simulink model "Loss_3Phase3Level_Inverter"  (Simulink 7.9)
settings: Solver=FixedStepDiscrete  StartTime=0.0  StopTime=12  FixedStep=Ts_Power  RelTol=1e-3
PreLoadFcn:
  | Ts_Power=5e-6
  | Ts_Control=50e-6
undefined symbols (not defined in the file or in its folder): D1, Delta
libraries: powerlib x23, powerlib_extras x21, fl_lib x12, LossModelib x3, nesl_utility x3, simulink x1
settings Model: Creator=Proprietaire  LastModifiedBy=at4494  SimulationMode=accelerator
settings DataIOCC: SaveOutput=off  SaveTime=off
settings OptimizationCC: EfficientMapNaN2IntZero=off
settings HardwareCC: TargetIntDivRoundTo=Zero  TargetEndianess=LittleEndian  TargetHWDeviceType=MATLAB Host  ProdEqTarget=off
settings CodeAppCC: MaxIdLength=128
settings GRTTargetCC: CombineOutputUpdateFcns=off  GRTInterface=on

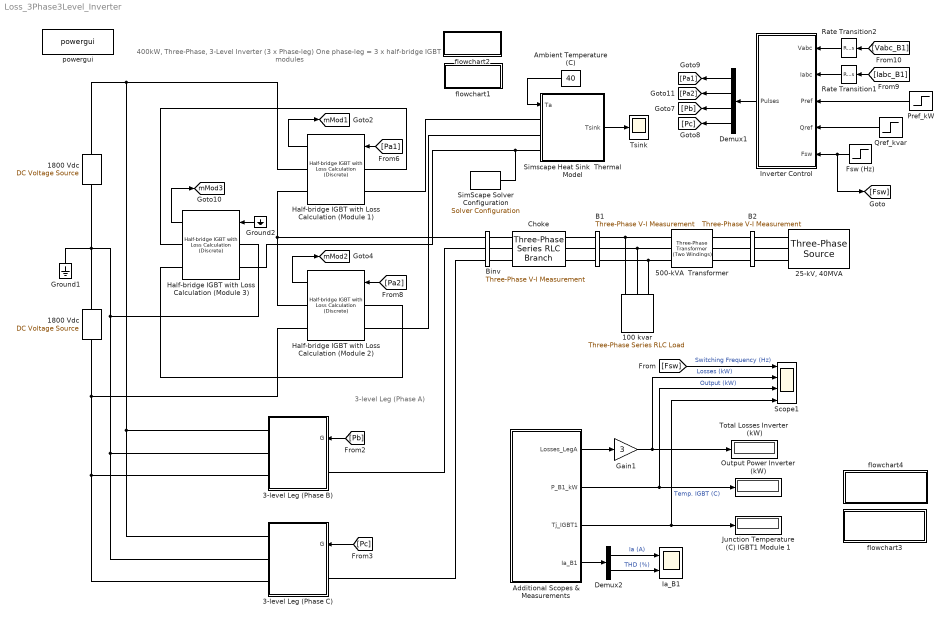
== system Loss_3Phase3Level_Inverter ==
  note: 400kW, Three-Phase, 3-Level Inverter (3 x Phase-leg)
      | One phase-leg = 3 x half-bridge IGBT modules
  note: 3-level Leg
      | (Phase A)
  100 kvar : powerlib/Elements/Three-Phase Series RLC Load  LConnTagsString=A|B|C  Configuration=Y (grounded)  NominalVoltage=2200  NominalFrequency=50  ActivePower=100e3/100  InductivePower=0  CapacitivePower=100e3  Measurements=None  LoadType=constant Z
  1800 Vdc : powerlib/Electrical Sources/DC Voltage Source  Description=source block  Amplitude=1800  Measurements=None
      settings: AttributesFormatString=\n
  "1800 Vdc " : powerlib/Electrical Sources/DC Voltage Source  Description=source block  Amplitude=1800  Measurements=None
      settings: AttributesFormatString=\n
  "25-kV, 40MVA" : powerlib/Electrical Sources/Three-Phase Source  Voltage=25e3*0.99  PhaseAngle=0  Frequency=50  InternalConnection=Yg  SpecifyImpedance=on  Resistance=0.8929  Inductance=16.58e-3  ShortCircuitLevel=40e6  BaseVoltage=25e3  XRratio=7  BusType=swing  Pref=0  Qref=0  Qmin=-inf  Qmax=inf
  3-level Leg (Phase B) : Subsystem
      mask Display:
      | dX=0.02-0.1;
      | dY=0.05-0.34;
      | K=1.4;
      | plot(([0.22 0.292 0.292]+dX)*K,([0.575 0.575 0.685]+dY)*K)
      | %plot([0.19 0.292 0.292]+dX,[0.195 0.195 0.305]+dY)
      | %plot([0.476 0.794]+dX,[0.455 0.455]+dY)
      | plot(([0.476 0.476 0.346 0.346 0.346 0.346 0.476 0.476]+dX)*K,([0.850 0.732 0.680 0.723 0.546 0.622 0.575 0.455 ]+dY)*K)
      | patch(([0.476 0.427 0.415 0.476]+dX)*K,([0.576 0.610 0.576 0.576]+dY)*K)
      | %
      | %plot([0.476 0.476 0.346 0.346 0.346 0.346 0.476 0.476]+dX,[0.850 0.732 0.680 0.723 0.546 0.622 0.575 0.455 ]-0.385+dY)
      | %patch([0.476 0.427 0.415 0.476]+dX,[0.576 0.610 0.576 0.576]-0.385+dY)
      | %
      | plot(([0.614 0.614 0.476]+dX)*K,([0.776 0.507 0.507]+dY)*K)
      | plot(([0.614 0.476]+dX)*K,([0.776 0.776]+dY)*K)
      | plot(([0.577 0.650]+dX)*K,([0.679 0.679]+dY)*K)
      | patch(([0.577 0.650  0.614 0.577]+dX)*K,([0.619 0.619 0.679 0.619]+dY)*K)
      | %
      | %plot([0.614 0.614 0.476]+dX,[0.776 0.507 0.507]-0.385+dY)
      | %plot([0.614 0.476]+dX,[0.776 0.776]-0.385+dY)
      | %plot([0.577 0.650]+dX,[0.679 0.679]-0.385+dY)
      | %patch([0.577 0.650  0.614 0.577]+dX,[0.619 0.619 0.679 0.619]-0.385+dY)
      | %
      | port_label('RConn', 1,'+');
      | port_label('RConn', 2,'N');
      | port_label('RConn', 3,'-');
      | port_label('LConn', 1,'B');
      | color('blue');
      | port_label('input', 1,'G');
  3-level Leg (Phase C) : Subsystem
      mask Display:
      | dX=0.02-0.1;
      | dY=0.05-0.34;
      | K=1.4;
      | plot(([0.22 0.292 0.292]+dX)*K,([0.575 0.575 0.685]+dY)*K)
      | %plot([0.19 0.292 0.292]+dX,[0.195 0.195 0.305]+dY)
      | %plot([0.476 0.794]+dX,[0.455 0.455]+dY)
      | plot(([0.476 0.476 0.346 0.346 0.346 0.346 0.476 0.476]+dX)*K,([0.850 0.732 0.680 0.723 0.546 0.622 0.575 0.455 ]+dY)*K)
      | patch(([0.476 0.427 0.415 0.476]+dX)*K,([0.576 0.610 0.576 0.576]+dY)*K)
      | %
      | %plot([0.476 0.476 0.346 0.346 0.346 0.346 0.476 0.476]+dX,[0.850 0.732 0.680 0.723 0.546 0.622 0.575 0.455 ]-0.385+dY)
      | %patch([0.476 0.427 0.415 0.476]+dX,[0.576 0.610 0.576 0.576]-0.385+dY)
      | %
      | plot(([0.614 0.614 0.476]+dX)*K,([0.776 0.507 0.507]+dY)*K)
      | plot(([0.614 0.476]+dX)*K,([0.776 0.776]+dY)*K)
      | plot(([0.577 0.650]+dX)*K,([0.679 0.679]+dY)*K)
      | patch(([0.577 0.650  0.614 0.577]+dX)*K,([0.619 0.619 0.679 0.619]+dY)*K)
      | %
      | %plot([0.614 0.614 0.476]+dX,[0.776 0.507 0.507]-0.385+dY)
      | %plot([0.614 0.476]+dX,[0.776 0.776]-0.385+dY)
      | %plot([0.577 0.650]+dX,[0.679 0.679]-0.385+dY)
      | %patch([0.577 0.650  0.614 0.577]+dX,[0.619 0.619 0.679 0.619]-0.385+dY)
      | %
      | port_label('RConn', 1,'+');
      | port_label('RConn', 2,'N');
      | port_label('RConn', 3,'-');
      | port_label('LConn', 1,'C');
      | color('blue');
      | port_label('input', 1,'G');
  500-kVA  Transformer : powerlib/Elements/Three-Phase Transformer (Two Windings)  Winding1Connection=Yg  UNITS=pu  NominalPower=[ 500e3 , 50 ]  Winding1=[ 25e3 , 0.001 , 0.025 ]  Winding2Connection=Delta (D1)  Winding2=[ 2200, 0.001 , 0.025 ]  SetSaturation=off  Rm=500  Lm=500  Saturation=[ 0,0 ; 0.0024,1.2 ; 1.0,1.52 ]  Hysteresis=off  DataFile='hysteresis'  SetInitialFlux=off  InitialFluxes=[ 0.8 , -0.8 , 0.7 ]  Measurements=None  MoreParameters=off  BreakLoop=off  DataType=off  TransfoNumber=1
  Additional Scopes & Measurements : Subsystem
  Ambient Temperature (C) : Constant  Value=40
  B1 : powerlib/Measurements/Three-Phase V-I Measurement  VoltageMeasurement=phase-to-ground  SetLabelV=on  LabelV=Vabc_B1  Vpu=off  VpuLL=off  CurrentMeasurement=yes  SetLabelI=on  LabelI=Iabc_B1  Ipu=off  Pbase=100e6  Vbase=500e3  OutputType=Complex  PhasorSimulation=off  PSBequivalent=0
  B2 : powerlib/Measurements/Three-Phase V-I Measurement  VoltageMeasurement=phase-to-ground  SetLabelV=on  LabelV=Vabc_B2  Vpu=off  VpuLL=off  CurrentMeasurement=yes  SetLabelI=on  LabelI=Iabc_B2  Ipu=off  Pbase=100e6  Vbase=500e3  OutputType=Complex  PhasorSimulation=off  PSBequivalent=0
  Binv : powerlib/Measurements/Three-Phase V-I Measurement  VoltageMeasurement=phase-to-ground  SetLabelV=on  LabelV=Vabc_Binv  Vpu=off  VpuLL=off  CurrentMeasurement=yes  SetLabelI=on  LabelI=Iabc_Binv  Ipu=off  Pbase=100e6  Vbase=500e3  OutputType=Complex  PhasorSimulation=off  PSBequivalent=0
  Choke : powerlib/Elements/Three-Phase Series RLC Branch  LConnTagsString=A|B|C  RConnTagsString=A|B|C  BranchType=RL  Resistance=15e-3  Inductance=5e-3  Capacitance=1e-6  Measurements=None
  Demux1 : Demux  Outputs=[ 2 2 4 4 ]
  Demux2 : Demux  Outputs=2
  Fsw (Hz) : Step  Time=5  Before=17*50  After=37*50  SampleTime=Ts_Control
  Gain1 : Gain  Gain=3
  Ground1 : powerlib/Elements/Ground  LConnTagsString=a
  Ground2 : Ground
  Half-bridge IGBT with Loss Calculation (Module 1) : LossModelib/Half-bridge IGBT with Loss Calculation (Discrete)  Ron=1e-3  IGBT_Type=ABB: Half-Bridge IGBT 3300V/250A  PlotSpec_IGBT_On=off  ShowDataSheet_IGBT_On=off  Diode_Type=ABB: Half-Bridge IGBT 3300V/250A  PlotSpec_Diode_On=off  ShowDataSheet_Diode_On=off  Tj_Init=123  PulseDuration=5e-6  Ts_Simscape=Ts_Control  Ts=Ts_Power
  Half-bridge IGBT with Loss Calculation (Module 2) : LossModelib/Half-bridge IGBT with Loss Calculation (Discrete)  Ron=1e-3  IGBT_Type=ABB: Half-Bridge IGBT 3300V/250A  PlotSpec_IGBT_On=off  ShowDataSheet_IGBT_On=off  Diode_Type=ABB: Half-Bridge IGBT 3300V/250A  PlotSpec_Diode_On=off  ShowDataSheet_Diode_On=off  Tj_Init=123  PulseDuration=5e-6  Ts_Simscape=Ts_Control  Ts=Ts_Power
  Half-bridge IGBT with Loss Calculation (Module 3) : LossModelib/Half-bridge IGBT with Loss Calculation (Discrete)  Ron=1e-3  IGBT_Type=ABB: Half-Bridge IGBT 3300V/250A  PlotSpec_IGBT_On=off  ShowDataSheet_IGBT_On=off  Diode_Type=ABB: Half-Bridge IGBT 3300V/250A  PlotSpec_Diode_On=off  ShowDataSheet_Diode_On=off  Tj_Init=123  PulseDuration=5e-6  Ts_Simscape=Ts_Control  Ts=Ts_Power
  Ia_B1 : Scope  NumInputPorts=2
      settings: TimeRange=12  YMin=-300~10  YMax=300~30  SaveName=psb1phPWM2_str3  MaxDataPoints=500000
  Inverter Control : Subsystem  mask(Inverter Control         ){nom=[ 500e3  50 ], Vnom=2200, Vnom_dc=2*1800, RLchoke=[15e-3  5e-3  ], K_PQreg=[ 0.2  60 ], K_Ireg=[0.3 20], Ts=Ts_Control}
      mask prompts: nom "Nominal power and frequency [ Pnom(VA)  Fnom(Hz) ]:"; Vnom "Nominal voltage (Vrms LL):"; Vnom_dc "Nominal DC bus voltage (V):"; RLchoke "Choke impedance [ R(ohm) L(H) ]"; K_PQreg "PQ regulator gains [ Kp  Ki ]:"; K_Ireg "Current regulator gains [ Kp  Ki ]:"; Ts "Sample time"
      mask init:
      | Pnom=nom(1);
      | Fnom=nom(2);
      | Zbase=Vnom^2/Pnom;
      | Rtot_pu= RLchoke(1)/Zbase;
      | Ltot_pu= RLchoke(2)/(Zbase/(2*pi*Fnom));
      | Kp_PQreg=K_PQreg(1);
      | Ki_PQreg=K_PQreg(2);
      | Kp_Ireg=K_Ireg(1);
      | Ki_Ireg=K_Ireg(2);
      | Vdc_ref=Vnom_dc;
  Junction Temperature (C) IGBT1 Module 1 : Display
      settings: Format=bank  Decimation=1000
  Output Power Inverter (kW) : Display
      settings: Format=bank  Decimation=1000
  Pref_kW : Step  Time=5.1  Before=372  After=211  SampleTime=Ts_Control
  Qref_kvar : Step  Time=5.1  Before=-sqrt(372^2*(1/(0.85)^2 - 1))  After=-sqrt(211^2*(1/(0.85)^2 - 1))  SampleTime=Ts_Control
  Rate Transition1 : RateTransition  OutPortSampleTime=Ts_Control
  Rate Transition2 : RateTransition  OutPortSampleTime=Ts_Control
  Scope1 : Scope  NumInputPorts=4
      settings: TimeRange=12  YMin=600~2~100~115  YMax=2000~4~500~135  SaveName=psb1phPWM2_str1  MaxDataPoints=500000  Decimation=10
  SimScape Solver Configuration : nesl_utility/Solver Configuration  PhysicalDomain=network_engine_domain  LeftPortType=input  RightPortType=generic  SubClassName=solver  UseCustomDae=off  DoDC=off  ResidualTolerance=1e-9  UseLocalSolver=on  LocalSolverChoice=NE_TRAPEZOIDAL_ADVANCER  LocalSolverSampleTime=Ts_Control  DoFixedCost=off  MaxNonlinIter=2  MaxModeIter=1  LinearAlgebra=Sparse  Accelerate=off  Profile=off  UseLocalSampling=off  DelaysMemoryBudget=1024
  Simscape Heat Sink  Thermal Model : Subsystem  mask(Simscape Thermal model (2-cell Cauer network)){Rth=[ 0.02  0.072 ], Cth=[ 1  5 ]/10, Tinit=123}
      mask prompts: Rth "Thermal resistances  [case-to-sink  sink-to-ambient ] (K/W):"; Cth "Thermal capacitances  [case  sink ] (J/K):"; Tinit "Initial temperature (degrees Celsisus)"
  Total Losses Inverter (kW) : Display
      settings: Format=bank  Decimation=1000
  Tsink : Scope
      settings: TimeRange=12  YMin=101.4492375546095  YMax=109.4893107691547  SaveName=psb1phPWM2_str6  MaxDataPoints=500000  Decimation=100
  flowchart1 : Subsystem
      settings: OpenFcn=winopen('ABB_PhaseLegModule_PCIM_12_408.pdf');
      mask Display: disp('Reference\nDocument')
  flowchart2 : Subsystem
      settings: OpenFcn=winopen('Loss_3Phase3Level_Inverter_Help.pdf');
      mask Display: disp('Help')
  flowchart3 : Subsystem
      settings: OpenFcn=plot_FFTresults
      mask Display: disp('Plot\nFFT Comparison')
  flowchart4 : Subsystem
      settings: OpenFcn=plot_OutputPower_vs_SwitchingFrequency
      mask Display: disp('Plot\n OutputPower vs.\nSwitching Frequency')
  powergui : powerlib/powergui  Priority=1  SimulationMode=Discrete  SolverType=Tustin  SampleTime=Ts_Power  frequency=60  SPID=off  DisableSnubberDevices=off  DisableRonSwitches=off  DisableVfSwitches=off  SwTol=0  Interpol=off  DisplayEquations=off  FunctionMessages=off  frequencyindice=0  Pbase=100e6  ErrMax=1e-4  Iterations=50  UnitsV=kV  UnitsW=MW  echomessages=off  HookPort=off  EnableUseOfTLC=off  x0status=blocks  RestoreLinks=warning  ResistiveCurrentMeasurement=off  Ylog=off  Xlog=on  ShowGrid=off  save=off  variable=ZData  structure=VIabc_B1  ZoomFFT=off  StartTime=4  cycles=3  DisplayStyle=1  fundamental=50  FreqAxis=on  MaxFrequency=2500  frequencyindicesteady=1  display=off  methode=off
  tag scope: mMod1=global, mMod2=global, mMod3=global
  wires:
  [Pb] -> 3-level Leg (Phase B)/1(G)
  Ambient Temperature (C)/1 -> Simscape Heat Sink  Thermal Model/1(Ta)
  [Pc] -> 3-level Leg (Phase C)/1(G)
  Additional Scopes & Measurements/1(Losses_LegA) -> Gain1/1
  [Vabc_B1] -> Rate Transition2/1
  [Iabc_B1] -> Rate Transition1/1
  Demux1/1 -> [Pa1]
  Demux1/2 -> [Pa2]
  Demux1/4 -> [Pc]
  Demux1/3 -> [Pb]
  Inverter Control/1(Pulses) -> Demux1/1
  Pref_kW/1 -> Inverter Control/3(Pref)
  Qref_kvar/1 -> Inverter Control/4(Qref)
  Additional Scopes & Measurements/2(P_B1_kW) -> Output Power Inverter (kW)/1, Scope1/3  "Output (kW)"
  Fsw (Hz)/1 -> Inverter Control/5(Fsw), [Fsw]
  Rate Transition1/1 -> Inverter Control/2(Iabc)
  Rate Transition2/1 -> Inverter Control/1(Vabc)
  Simscape Heat Sink  Thermal Model/1(Tsink) -> Tsink/1
  Half-bridge IGBT with Loss Calculation (Module 3)/1 -> [mMod3]
  Half-bridge IGBT with Loss Calculation (Module 2)/1 -> [mMod2]
  Ground2/1 -> Half-bridge IGBT with Loss Calculation (Module 3)/1
  [Pa1] -> Half-bridge IGBT with Loss Calculation (Module 1)/1
  [Pa2] -> Half-bridge IGBT with Loss Calculation (Module 2)/1
  Half-bridge IGBT with Loss Calculation (Module 1)/1 -> [mMod1]
  Additional Scopes & Measurements/3(Tj_IGBT1) -> Junction Temperature (C) IGBT1 Module 1/1, Scope1/4  "Temp. IGBT (C)"
  Gain1/1 -> Total Losses Inverter (kW)/1, Scope1/2  "Losses (kW)"
  [Fsw] -> Scope1/1  "Switching Frequency (Hz)"
  Demux2/1 -> Ia_B1/1  "Ia (A)"
  Demux2/2 -> Ia_B1/2  "THD (%)"
  Additional Scopes & Measurements/4(Ia_B1) -> Demux2/1
  connections:
  Half-bridge IGBT with Loss Calculation (Module 3)/LConn2 -- SimScape Solver Configuration/RConn1 -- Simscape Heat Sink  Thermal Model/LConn3
  Choke/RConn1 -- B1/LConn1
  Choke/RConn2 -- B1/LConn2
  Choke/RConn3 -- B1/LConn3
  "25-kV, 40MVA"/RConn1 -- B2/RConn1
  "25-kV, 40MVA"/RConn2 -- B2/RConn2
  "25-kV, 40MVA"/RConn3 -- B2/RConn3
  Choke/LConn1 -- Binv/RConn1
  Choke/LConn2 -- Binv/RConn2
  Choke/LConn3 -- Binv/RConn3
  Binv/LConn2 -- 3-level Leg (Phase B)/LConn1
  Binv/LConn3 -- 3-level Leg (Phase C)/LConn1
  500-kVA  Transformer/RConn1 -- B1/RConn1 -- 100 kvar/LConn1
  500-kVA  Transformer/RConn2 -- B1/RConn2 -- 100 kvar/LConn2
  B1/RConn3 -- 500-kVA  Transformer/RConn3 -- 100 kvar/LConn3
  500-kVA  Transformer/LConn1 -- B2/LConn1
  500-kVA  Transformer/LConn2 -- B2/LConn2
  500-kVA  Transformer/LConn3 -- B2/LConn3
  Half-bridge IGBT with Loss Calculation (Module 1)/RConn2 -- Binv/LConn1 -- Half-bridge IGBT with Loss Calculation (Module 2)/RConn1
  Half-bridge IGBT with Loss Calculation (Module 3)/LConn1 -- 3-level Leg (Phase B)/RConn2 -- 3-level Leg (Phase C)/RConn2 -- 1800 Vdc/RConn1 -- Ground1/LConn1 -- "1800 Vdc "/LConn1
  Simscape Heat Sink  Thermal Model/LConn1 -- Half-bridge IGBT with Loss Calculation (Module 1)/LConn2
  Half-bridge IGBT with Loss Calculation (Module 1)/RConn1 -- 3-level Leg (Phase B)/RConn1 -- 3-level Leg (Phase C)/RConn1 -- "1800 Vdc "/RConn1
  Half-bridge IGBT with Loss Calculation (Module 2)/RConn2 -- 3-level Leg (Phase B)/RConn3 -- 3-level Leg (Phase C)/RConn3 -- 1800 Vdc/LConn1
  Half-bridge IGBT with Loss Calculation (Module 3)/RConn1 -- Half-bridge IGBT with Loss Calculation (Module 1)/LConn1
  Half-bridge IGBT with Loss Calculation (Module 2)/LConn1 -- Half-bridge IGBT with Loss Calculation (Module 3)/RConn2
  Half-bridge IGBT with Loss Calculation (Module 2)/LConn2 -- Simscape Heat Sink  Thermal Model/LConn2

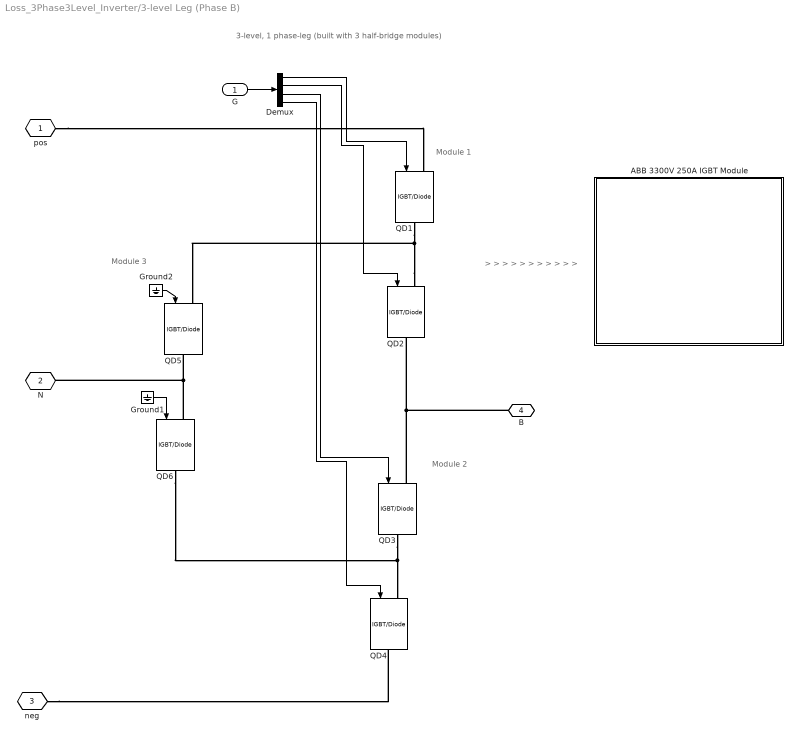
== system Loss_3Phase3Level_Inverter/3-level Leg (Phase B) ==
  note: Module 3
  note: Module 2
  note: 3-level, 1 phase-leg
      |  (built with 3 half-bridge modules)
  note: Module 1
  note: > > > > > > > > > > >
  G : Inport  PortDimensions=4
  ABB 3300V 250A IGBT Module : Subsystem
      mask Display: image(imread('Picture_IGBT_Module.jpg'))
  Demux : Demux
  Ground1 : Ground
  Ground2 : Ground
  QD{1..6} (6 alike) : powerlib/Power Electronics/IGBT//Diode  Ron=1e-3  Rs=1e5  Cs=inf  Measurements=off
  pos : PMIOPort  Port=1  Side=Right
  N : PMIOPort  Port=2  Side=Right
  neg : PMIOPort  Port=3  Side=Right
  B : PMIOPort  Port=4  Side=Left
  wires:
  Demux/4 -> QD4/1
  Demux/3 -> QD3/1
  Ground1/1 -> QD6/1
  Ground2/1 -> QD5/1
  G/1 -> Demux/1
  Demux/1 -> QD1/1
  Demux/2 -> QD2/1
  connections:
  N/RConn1 -- QD6/LConn1 -- QD5/RConn1
  QD3/RConn1 -- QD4/LConn1 -- QD6/RConn1
  QD2/LConn1 -- QD1/RConn1 -- QD5/LConn1
  pos/RConn1 -- QD1/LConn1
  QD3/LConn1 -- QD2/RConn1 -- B/RConn1
  neg/RConn1 -- QD4/RConn1

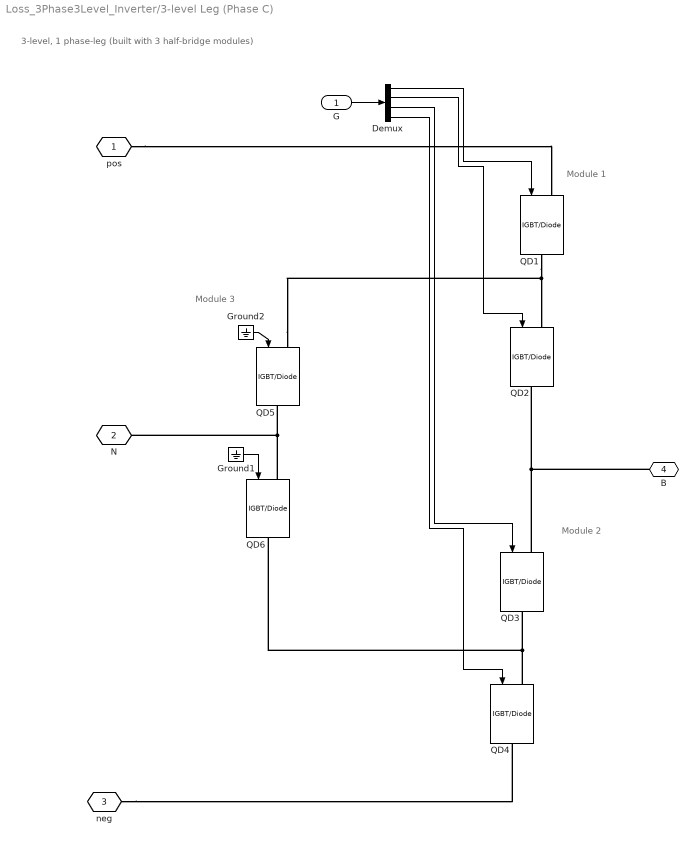
== system Loss_3Phase3Level_Inverter/3-level Leg (Phase C) ==
  note: Module 1
  note: 3-level, 1 phase-leg
      |  (built with 3 half-bridge modules)
  note: Module 2
  note: Module 3
  G : Inport  PortDimensions=4
  Demux : Demux
  Ground1 : Ground
  Ground2 : Ground
  QD{1..6} (6 alike) : powerlib/Power Electronics/IGBT//Diode  Ron=1e-3  Rs=1e5  Cs=inf  Measurements=off
  pos : PMIOPort  Port=1  Side=Right
  N : PMIOPort  Port=2  Side=Right
  neg : PMIOPort  Port=3  Side=Right
  B : PMIOPort  Port=4  Side=Left
  wires:
  Demux/2 -> QD2/1
  Demux/1 -> QD1/1
  G/1 -> Demux/1
  Ground2/1 -> QD5/1
  Ground1/1 -> QD6/1
  Demux/3 -> QD3/1
  Demux/4 -> QD4/1
  connections:
  neg/RConn1 -- QD4/RConn1
  B/RConn1 -- QD2/RConn1 -- QD3/LConn1
  pos/RConn1 -- QD1/LConn1
  QD5/LConn1 -- QD2/LConn1 -- QD1/RConn1
  QD4/LConn1 -- QD3/RConn1 -- QD6/RConn1
  QD6/LConn1 -- N/RConn1 -- QD5/RConn1

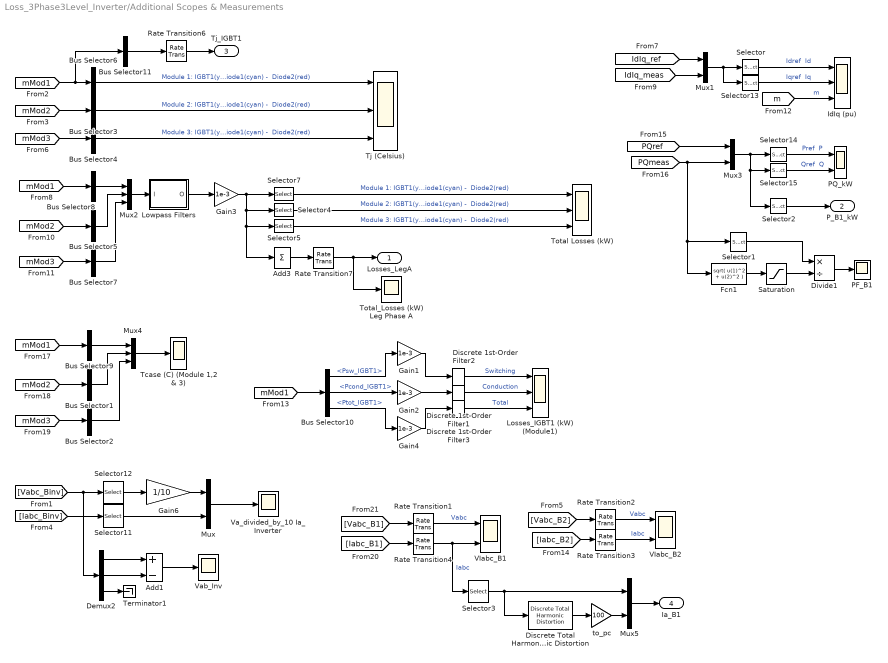
== system Loss_3Phase3Level_Inverter/Additional Scopes & Measurements ==
  Add1 : Sum  Inputs=+-
  Add3 : Sum  Inputs=+
  Bus Selector1 : BusSelector  OutputSignals=Tcase  OutputAsBus=on
  Bus Selector10 : BusSelector  OutputSignals=Psw_IGBT1,Pcond_IGBT1,Ptot_IGBT1
  Bus Selector11 : BusSelector  OutputSignals=Tj_IGBT1  OutputAsBus=on
  Bus Selector2 : BusSelector  OutputSignals=Tcase  OutputAsBus=on
  Bus Selector3 : BusSelector  OutputSignals=Tj_IGBT1,Tj_IGBT2,Tj_Diode1,Tj_Diode2  OutputAsBus=on
  Bus Selector4 : BusSelector  OutputSignals=Tj_IGBT1,Tj_IGBT2,Tj_Diode1,Tj_Diode2  OutputAsBus=on
  Bus Selector5 : BusSelector  OutputSignals=Ptot_IGBT1,Ptot_IGBT2,Ptot_Diode1,Ptot_Diode2  OutputAsBus=on
  Bus Selector6 : BusSelector  OutputSignals=Tj_IGBT1,Tj_IGBT2,Tj_Diode1,Tj_Diode2  OutputAsBus=on
  Bus Selector7 : BusSelector  OutputSignals=Ptot_IGBT1,Ptot_IGBT2,Ptot_Diode1,Ptot_Diode2  OutputAsBus=on
  Bus Selector8 : BusSelector  OutputSignals=Ptot_IGBT1,Ptot_IGBT2,Ptot_Diode1,Ptot_Diode2  OutputAsBus=on
  Bus Selector9 : BusSelector  OutputSignals=Tcase  OutputAsBus=on
  Demux2 : Demux  Outputs=3
  Discrete 1st-Order Filter1 : powerlib_extras/Discrete  Control Blocks/Discrete 1st-Order Filter  FilterType=Lowpass  Tc=100e-3  Ts=Ts_Power  Initialize=off  Vac_Init=[0.8 -25 60]  Vdc_Init=-0.4  PlotResponse=off  param1=[1 500 0.1]
  Discrete 1st-Order Filter2 : powerlib_extras/Discrete  Control Blocks/Discrete 1st-Order Filter  FilterType=Lowpass  Tc=100e-3  Ts=Ts_Power  Initialize=off  Vac_Init=[0.8 -25 60]  Vdc_Init=-0.4  PlotResponse=off  param1=[1 500 0.1]
  Discrete 1st-Order Filter3 : powerlib_extras/Discrete  Control Blocks/Discrete 1st-Order Filter  FilterType=Lowpass  Tc=100e-3  Ts=Ts_Power  Initialize=off  Vac_Init=[0.8 -25 60]  Vdc_Init=-0.4  PlotResponse=off  param1=[1 500 0.1]
  Discrete Total Harmonic Distortion : powerlib_extras/Discrete Measurements/Discrete Total Harmonic Distortion  Freq=50  Ts=Ts_Control
  Divide1 : Product  Inputs=*/
  Fcn1 : Fcn  Expr=sqrt( u(1)^2 + u(2)^2 )
  Gain{1..4} (4 alike) : Gain  Gain=1e-3
  Gain6 : Gain  Gain=1/10
  IdIq (pu) : Scope  NumInputPorts=3
      settings: TimeRange=12  YMin=0~0~0.7000000000000001  YMax=1.4~1.4~1.2  SaveName=Vab_Load  MaxDataPoints=500000
  Losses_IGBT1 (kW) (Module1) : Scope  NumInputPorts=3
      settings: TimeRange=12  YMin=0~0~0  YMax=0.4~0.1~0.4  SaveName=Va_Load  MaxDataPoints=500000  Decimation=100
  Lowpass Filters : Subsystem  mask(12 x First-Order Lowpass Filters){Tc=100e-3, Ts=Ts_Power}
      mask prompts: Tc "Time constant (s):"; Ts "Sample time (s):"
  Mux : Mux  Inputs=2
  Mux1 : Mux  Inputs="[ 2  2 ]"
  Mux2 : Mux  Inputs=3
  Mux3 : Mux  Inputs="[ 2  2 ]"
  Mux4 : Mux  Inputs=3
  Mux5 : Mux  Inputs=2
  PF_B1 : Scope
      settings: TimeRange=12  YMin=0.8180348878604487  YMax=0.8857030971876113  SaveName=Va_Load5  MaxDataPoints=500000
  PQ_kW : Scope  NumInputPorts=2
      settings: TimeRange=12  YMin=0~-400  YMax=500~100  SaveName=Vab_Load2  MaxDataPoints=500000
  Rate Transition{1..4,6..7} (6 alike) : RateTransition  OutPortSampleTime=Ts_Control
  Saturation : Saturate  UpperLimit=inf  LowerLimit=eps
  Selector : Selector  InputPortWidth=4  IndexOptions=Index vector (dialog)  Indices=[1 3]  OutputSizes=1
  Selector1 : Selector  InputPortWidth=2  IndexOptions=Index vector (dialog)  Indices=[1]  OutputSizes=1
  Selector11 : Selector  InputPortWidth=3  IndexOptions=Index vector (dialog)  Indices=[1]  OutputSizes=1
  Selector12 : Selector  InputPortWidth=3  IndexOptions=Index vector (dialog)  Indices=[1]  OutputSizes=1
  Selector13 : Selector  InputPortWidth=4  IndexOptions=Index vector (dialog)  Indices=[1 3]  OutputSizes=1
  Selector14 : Selector  InputPortWidth=4  IndexOptions=Index vector (dialog)  Indices=[1 3]  OutputSizes=1
  Selector15 : Selector  InputPortWidth=4  IndexOptions=Index vector (dialog)  Indices=[2 4]  OutputSizes=1
  Selector2 : Selector  InputPortWidth=4  IndexOptions=Index vector (dialog)  Indices=[3]  OutputSizes=1
  Selector3 : Selector  InputPortWidth=3  IndexOptions=Index vector (dialog)  Indices=[1]  OutputSizes=1
  Selector4 : Selector  InputPortWidth=12  IndexOptions=Index vector (dialog)  Indices=[1 2 3 4]+4  OutputSizes=1
  Selector5 : Selector  InputPortWidth=12  IndexOptions=Index vector (dialog)  Indices=[1 2 3 4]+8  OutputSizes=1
  Selector7 : Selector  InputPortWidth=12  IndexOptions=Index vector (dialog)  Indices=[1 2 3 4]  OutputSizes=1
  Tcase (C) (Module 1,2 & 3) : Scope
      settings: TimeRange=12  YMin=100  YMax=120  SaveName=psb1phPWM2_str2  MaxDataPoints=500000  Decimation=100
  Terminator1 : Terminator
  Tj (Celsius) : Scope  NumInputPorts=3
      settings: TimeRange=12  YMin=105~105~105  YMax=135~135~135  SaveName=psb1phPWM2_str  MaxDataPoints=500000  Decimation=100
  "Total Losses (kW) " : Scope  NumInputPorts=3
      settings: TimeRange=12  YMin=0~0~0  YMax=0.4~0.4~0.14  SaveName=Losses_Scope  MaxDataPoints=500000  Decimation=100
  Total_Losses (kW) Leg Phase A : Scope
      settings: TimeRange=12  YMin=0  YMax=1.4  SaveName=Va_Load6  MaxDataPoints=500000  Decimation=10
  VIabc_B1 : Scope  NumInputPorts=2
      settings: TimeRange=12  YMin=-2500~-504.4510385756676  YMax=2500~459.9406528189911  SaveName=VIabc_B1  MaxDataPoints=500000
  VIabc_B2 : Scope  NumInputPorts=2
      settings: YMin=-25000~-20  YMax=25000~25  SaveName=VIabc_B2  MaxDataPoints=500000
  Va_divided_by_10 Ia_Inverter : Scope
      settings: YMin=-500  YMax=500  SaveName=psb1phPWM2_str5  MaxDataPoints=500000  Decimation=2
  Vab_Inv : Scope
      settings: TimeRange=0.08  YMin=-4000  YMax=4000  SaveName=Vab_Inv  MaxDataPoints=500000  Decimation=2
  to_pc : Gain  Gain=100
  Losses_LegA : Outport
  P_B1_kW : Outport  Port=2
  Tj_IGBT1 : Outport  Port=3
  Ia_B1 : Outport  Port=4
  wires:
  Mux/1 -> Va_divided_by_10 Ia_Inverter/1
  [mMod1] -> Bus Selector6/1, Bus Selector11/1
  [mMod2] -> Bus Selector3/1
  [mMod3] -> Bus Selector4/1
  [mMod1] -> Bus Selector8/1
  [mMod2] -> Bus Selector5/1
  [mMod3] -> Bus Selector7/1
  Mux2/1 -> Lowpass Filters/1(I)
  Selector7/1 -> "Total Losses (kW) "/1  "Module 1: IGBT1(yellow) -  IGBT2(magenta)  -  Diode1(cyan) -  Diode2(red)"
  Selector4/1 -> "Total Losses (kW) "/2  "Module 2: IGBT1(yellow) -  IGBT2(magenta)  -  Diode1(cyan) -  Diode2(red)"
  Selector5/1 -> "Total Losses (kW) "/3  "Module 3: IGBT1(yellow) -  IGBT2(magenta)  -  Diode1(cyan) -  Diode2(red)"
  Bus Selector8/1 -> Mux2/1
  Bus Selector5/1 -> Mux2/2
  Bus Selector7/1 -> Mux2/3
  Lowpass Filters/1(O) -> Gain3/1
  Gain3/1 -> Selector7/1, Add3/1, Selector5/1, Selector4/1
  Add3/1 -> Rate Transition7/1
  [Vabc_Binv] -> Selector12/1, Demux2/1
  [Iabc_Binv] -> Selector11/1
  Selector12/1 -> Gain6/1
  Selector11/1 -> Mux/2
  Gain6/1 -> Mux/1
  Fcn1/1 -> Saturation/1
  Selector1/1 -> Divide1/1
  Divide1/1 -> PF_B1/1
  [IdIq_ref] -> Mux1/1
  Saturation/1 -> Divide1/2
  Demux2/1 -> Add1/1
  Demux2/2 -> Add1/2
  Demux2/3 -> Terminator1/1
  Add1/1 -> Vab_Inv/1
  [mMod1] -> Bus Selector9/1
  [mMod2] -> Bus Selector1/1
  [mMod3] -> Bus Selector2/1
  Bus Selector9/1 -> Mux4/1
  Bus Selector1/1 -> Mux4/2
  Bus Selector2/1 -> Mux4/3
  Mux4/1 -> Tcase (C) (Module 1,2 & 3)/1
  [m] -> IdIq (pu)/3  "m"
  [IdIq_meas] -> Mux1/2
  Mux1/1 -> Selector/1, Selector13/1
  Selector/1 -> IdIq (pu)/1  "Idref  Id"
  Selector13/1 -> IdIq (pu)/2  "Iqref  Iq"
  [PQref] -> Mux3/1
  [PQmeas] -> Mux3/2, Selector1/1, Fcn1/1
  Mux3/1 -> Selector14/1, Selector15/1, Selector2/1
  Selector14/1 -> PQ_kW/1  "Pref  P"
  Selector15/1 -> PQ_kW/2  "Qref  Q"
  Selector2/1 -> P_B1_kW/1
  [Vabc_B1] -> Rate Transition1/1
  [Iabc_B1] -> Rate Transition4/1
  Rate Transition1/1 -> VIabc_B1/1  "Vabc"
  Rate Transition4/1 -> VIabc_B1/2, Selector3/1  "Iabc"
  [mMod1] -> Bus Selector10/1
  Bus Selector10/1 -> Gain1/1  "<Psw_IGBT1>"
  Bus Selector10/2 -> Gain2/1  "<Pcond_IGBT1>"
  Bus Selector10/3 -> Gain4/1  "<Ptot_IGBT1>"
  Discrete 1st-Order Filter2/1 -> Losses_IGBT1 (kW) (Module1)/1  "Switching"
  Rate Transition2/1 -> VIabc_B2/1  "Vabc"
  Rate Transition3/1 -> VIabc_B2/2  "Iabc"
  [Vabc_B2] -> Rate Transition2/1
  [Iabc_B2] -> Rate Transition3/1
  Bus Selector6/1 -> Tj (Celsius)/1  "Module 1: IGBT1(yellow) -  IGBT2(magenta)  -  Diode1(cyan) -  Diode2(red)"
  Bus Selector3/1 -> Tj (Celsius)/2  "Module 2: IGBT1(yellow) -  IGBT2(magenta)  -  Diode1(cyan) -  Diode2(red)"
  Bus Selector4/1 -> Tj (Celsius)/3  "Module 3: IGBT1(yellow) -  IGBT2(magenta)  -  Diode1(cyan) -  Diode2(red)"
  Discrete 1st-Order Filter1/1 -> Losses_IGBT1 (kW) (Module1)/2  "Conduction"
  Discrete 1st-Order Filter3/1 -> Losses_IGBT1 (kW) (Module1)/3  "Total"
  Gain1/1 -> Discrete 1st-Order Filter2/1
  Gain2/1 -> Discrete 1st-Order Filter1/1
  Gain4/1 -> Discrete 1st-Order Filter3/1
  Rate Transition6/1 -> Tj_IGBT1/1
  Bus Selector11/1 -> Rate Transition6/1
  Rate Transition7/1 -> Losses_LegA/1, Total_Losses (kW) Leg Phase A/1
  Discrete Total Harmonic Distortion/1 -> to_pc/1
  Selector3/1 -> Mux5/1, Discrete Total Harmonic Distortion/1
  Mux5/1 -> Ia_B1/1
  to_pc/1 -> Mux5/2

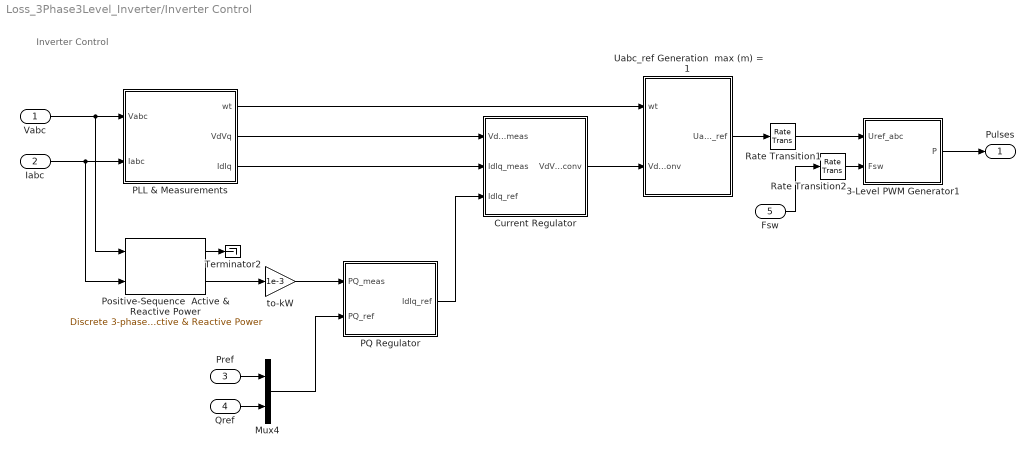
== system Loss_3Phase3Level_Inverter/Inverter Control ==
  note: Inverter Control
  Vabc : Inport  PortDimensions=3  SampleTime=Ts
  Iabc : Inport  Port=2  PortDimensions=3  SampleTime=Ts
  Pref : Inport  Port=3  PortDimensions=1  SampleTime=Ts
  Qref : Inport  Port=4  PortDimensions=1  SampleTime=Ts
  Fsw : Inport  Port=5  PortDimensions=1
  " Positive-Sequence  Active & Reactive Power" : powerlib_extras/Discrete Measurements/Discrete 3-phase  Positive-Sequence  Active & Reactive Power  Freq=Fnom  Par_Vinit=[100 10]  Par_Iinit=[1 1]  Ts=Ts
  3-Level PWM Generator1 : Subsystem  mask(Discrete 3-Phase, 3-Level, PWM Generator){Ts=Ts_Power}
      mask prompts: Ts "Sample time (s):"
      mask help:
      | Generate pulses for carrier-based Pulse Width Modulation (PWM) 3-Level, 3-Phase converters.
      | Input 1: Three-phase reference signals (Uref_abc)
      | Input 2: Switching frequency (Fsw)
      | Output: Vectorized output P contains the 12 pulses.  Look Under Mask to get a description of the pulse pattern.
  Current Regulator : Subsystem
  Mux4 : Mux  Inputs=2
  PLL & Measurements : Subsystem
  PQ Regulator : Subsystem
  Rate Transition1 : RateTransition  OutPortSampleTime=Ts_Power
  Rate Transition2 : RateTransition  OutPortSampleTime=Ts_Power
  Terminator2 : Terminator
  Uabc_ref Generation  max (m) = 1 : Subsystem
  to-kW : Gain  Gain=1e-3  SaturateOnIntegerOverflow=on  OutDataTypeStr=Inherit: Same as input  ParamDataTypeStr=Inherit: Same as input
  Pulses : Outport
  wires:
  Uabc_ref Generation  max (m) = 1/1(Uabc_ref) -> Rate Transition1/1
  Iabc/1 -> PLL & Measurements/2(Iabc), " Positive-Sequence  Active & Reactive Power"/2
  Vabc/1 -> PLL & Measurements/1(Vabc), " Positive-Sequence  Active & Reactive Power"/1
  PLL & Measurements/2(VdVq) -> Current Regulator/1(VdVq_meas)
  PLL & Measurements/3(IdIq) -> Current Regulator/2(IdIq_meas)
  Current Regulator/1(VdVq_conv) -> Uabc_ref Generation  max (m) = 1/2(VdVq_conv)
  PLL & Measurements/1(wt) -> Uabc_ref Generation  max (m) = 1/1(wt)
  Rate Transition1/1 -> 3-Level PWM Generator1/1(Uref_abc)
  " Positive-Sequence  Active & Reactive Power"/2 -> to-kW/1
  Pref/1 -> Mux4/1
  Qref/1 -> Mux4/2
  " Positive-Sequence  Active & Reactive Power"/1 -> Terminator2/1
  Mux4/1 -> PQ Regulator/2(PQ_ref)
  PQ Regulator/1(IdIq_ref) -> Current Regulator/3(IdIq_ref)
  to-kW/1 -> PQ Regulator/1(PQ_meas)
  Fsw/1 -> Rate Transition2/1
  3-Level PWM Generator1/1(P) -> Pulses/1
  Rate Transition2/1 -> 3-Level PWM Generator1/2(Fsw)

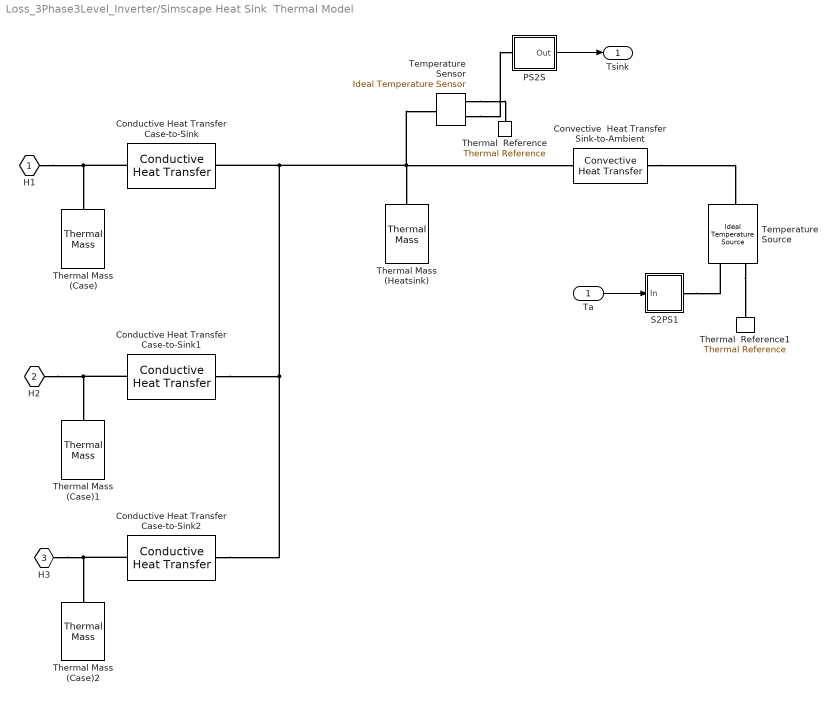
== system Loss_3Phase3Level_Inverter/Simscape Heat Sink  Thermal Model ==
  Ta : Inport
  Conductive Heat Transfer Case-to-Sink : fl_lib/Thermal/Thermal Elements/Conductive Heat Transfer  area=1 m^2  thickness=1 m  th_cond=1/Rth(1) W/(m*K)  Q_Log=off  T_Log=off  LocalVarNames=|Q|T  LocalVarDescs=|Q|T  LocalVarLogging=[0 0]
  Conductive Heat Transfer Case-to-Sink1 : fl_lib/Thermal/Thermal Elements/Conductive Heat Transfer  area=1 m^2  thickness=1 m  th_cond=1/Rth(1) W/(m*K)  Q_Log=off  T_Log=off  LocalVarNames=|Q|T  LocalVarDescs=|Q|T  LocalVarLogging=[0 0]
  Conductive Heat Transfer Case-to-Sink2 : fl_lib/Thermal/Thermal Elements/Conductive Heat Transfer  area=1 m^2  thickness=1 m  th_cond=1/Rth(1) W/(m*K)  Q_Log=off  T_Log=off  LocalVarNames=|Q|T  LocalVarDescs=|Q|T  LocalVarLogging=[0 0]
  Convective  Heat Transfer Sink-to-Ambient : fl_lib/Thermal/Thermal Elements/Convective Heat Transfer  area=1 m^2  heat_tr_coeff=1/Rth(2) W/(m^2 * K)  Q_Log=off  T_Log=off  LocalVarNames=|Q|T  LocalVarDescs=|Q|T  LocalVarLogging=[0 0]
  PS2S : Subsystem
  S2PS1 : Subsystem
  Temperature Sensor : fl_lib/Thermal/Thermal Sensors/Ideal Temperature Sensor  Qs_Log=off  Ts_Log=off  LocalVarNames=|Qs|Ts  LocalVarDescs=|Qs|Ts  LocalVarLogging=[0 0]
  Temperature Source : fl_lib/Thermal/Thermal Sources/Ideal Temperature Source  Q_Log=off  T_Log=off  LocalVarNames=|Q|T  LocalVarDescs=|Q|T  LocalVarLogging=[0 0]
  Thermal  Reference : fl_lib/Thermal/Thermal Elements/Thermal Reference  Q_Log=off  LocalVarNames=|Q  LocalVarDescs=|Q  LocalVarLogging=0
  Thermal  Reference1 : fl_lib/Thermal/Thermal Elements/Thermal Reference  Q_Log=off  LocalVarNames=|Q  LocalVarDescs=|Q  LocalVarLogging=0
  Thermal Mass (Case) : fl_lib/Thermal/Thermal Elements/Thermal Mass  mass=Cth(1) kg  sp_heat=1 J/kg/K  init_temp=Tinit K  Q_Log=off  LocalVarNames=|Q  LocalVarDescs=|Q  LocalVarLogging=0
  Thermal Mass (Case)1 : fl_lib/Thermal/Thermal Elements/Thermal Mass  mass=Cth(1) kg  sp_heat=1 J/kg/K  init_temp=Tinit K  Q_Log=off  LocalVarNames=|Q  LocalVarDescs=|Q  LocalVarLogging=0
  Thermal Mass (Case)2 : fl_lib/Thermal/Thermal Elements/Thermal Mass  mass=Cth(1) kg  sp_heat=1 J/kg/K  init_temp=Tinit K  Q_Log=off  LocalVarNames=|Q  LocalVarDescs=|Q  LocalVarLogging=0
  Thermal Mass (Heatsink) : fl_lib/Thermal/Thermal Elements/Thermal Mass  mass=Cth(2) kg  sp_heat=1 J/kg/K  init_temp=Tinit K  Q_Log=off  LocalVarNames=|Q  LocalVarDescs=|Q  LocalVarLogging=0
  H1 : PMIOPort  Port=1  Side=Left
  H2 : PMIOPort  Port=2  Side=Left
  H3 : PMIOPort  Port=3  Side=Left
  Tsink : Outport
  wires:
  PS2S/1(Out) -> Tsink/1
  Ta/1 -> S2PS1/1(In)
  connections:
  Temperature Sensor/RConn2 -- PS2S/LConn1
  Temperature Sensor/RConn1 -- Thermal  Reference/LConn1
  Conductive Heat Transfer Case-to-Sink1/RConn1 -- Temperature Sensor/LConn1 -- Thermal Mass (Heatsink)/LConn1 -- Convective  Heat Transfer Sink-to-Ambient/LConn1 -- Conductive Heat Transfer Case-to-Sink/RConn1 -- Conductive Heat Transfer Case-to-Sink2/RConn1
  Convective  Heat Transfer Sink-to-Ambient/RConn1 -- Temperature Source/LConn1
  S2PS1/RConn1 -- Temperature Source/RConn1
  Temperature Source/RConn2 -- Thermal  Reference1/LConn1
  Conductive Heat Transfer Case-to-Sink/LConn1 -- Thermal Mass (Case)/LConn1 -- H1/RConn1
  H2/RConn1 -- Thermal Mass (Case)1/LConn1 -- Conductive Heat Transfer Case-to-Sink1/LConn1
  H3/RConn1 -- Conductive Heat Transfer Case-to-Sink2/LConn1 -- Thermal Mass (Case)2/LConn1

== system Loss_3Phase3Level_Inverter/flowchart1 ==

== system Loss_3Phase3Level_Inverter/flowchart2 ==

== system Loss_3Phase3Level_Inverter/flowchart3 ==

== system Loss_3Phase3Level_Inverter/flowchart4 ==

== system Loss_3Phase3Level_Inverter/3-level Leg (Phase B)/ABB 3300V 250A IGBT Module ==

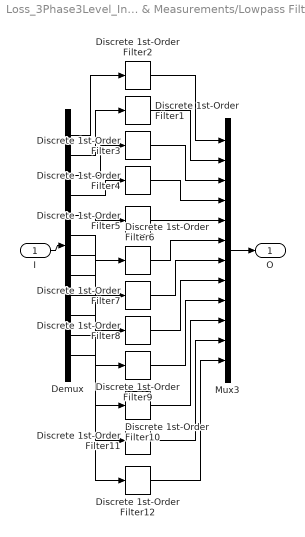
== system Loss_3Phase3Level_Inverter/Additional Scopes & Measurements/Lowpass Filters ==
  I : Inport
  Demux : Demux  Outputs=12
  Discrete 1st-Order Filter{1..12} (12 alike) : powerlib_extras/Discrete  Control Blocks/Discrete 1st-Order Filter  FilterType=Lowpass  Tc=Tc  Ts=Ts  Initialize=off  Vac_Init=[0.8 -25 60]  Vdc_Init=-0.4  PlotResponse=off  param1=[1 500 0.1]
  Mux3 : Mux  Inputs=12
  O : Outport
  wires:
  Demux/1 -> Discrete 1st-Order Filter2/1
  Demux/2 -> Discrete 1st-Order Filter1/1
  Demux/3 -> Discrete 1st-Order Filter3/1
  Demux/4 -> Discrete 1st-Order Filter4/1
  Demux/5 -> Discrete 1st-Order Filter5/1
  Demux/6 -> Discrete 1st-Order Filter6/1
  Demux/7 -> Discrete 1st-Order Filter7/1
  Demux/8 -> Discrete 1st-Order Filter8/1
  Demux/9 -> Discrete 1st-Order Filter9/1
  Demux/10 -> Discrete 1st-Order Filter10/1
  Demux/11 -> Discrete 1st-Order Filter11/1
  Demux/12 -> Discrete 1st-Order Filter12/1
  Discrete 1st-Order Filter2/1 -> Mux3/1
  Discrete 1st-Order Filter1/1 -> Mux3/2
  Discrete 1st-Order Filter3/1 -> Mux3/3
  Discrete 1st-Order Filter4/1 -> Mux3/4
  Discrete 1st-Order Filter5/1 -> Mux3/5
  Discrete 1st-Order Filter6/1 -> Mux3/6
  Discrete 1st-Order Filter7/1 -> Mux3/7
  Discrete 1st-Order Filter8/1 -> Mux3/8
  Discrete 1st-Order Filter9/1 -> Mux3/9
  Discrete 1st-Order Filter10/1 -> Mux3/10
  Discrete 1st-Order Filter11/1 -> Mux3/11
  Discrete 1st-Order Filter12/1 -> Mux3/12
  I/1 -> Demux/1
  Mux3/1 -> O/1

== system Loss_3Phase3Level_Inverter/Inverter Control/3-Level PWM Generator1 ==
  note: 3-phase State-to-Pulses Decoder
  note: --------------------------------------------------------------
  note: |
      | |
      | |
      | |
      | |
      | |
      | |
      | |
      | |
  note: 1
  note: 1
  note: 0
  note: 0
  note: -1
  note: 0
  note: 1
  note: 1
  note: 0
  note: 0
  note: Q4
  note: Q3
  note: Q2
  note: Q1
  note: 0
  note: 0
  note: 1
  note: 1
  note: Firing pulses
  note: 1
  note: State
  note: + Vdc --------------------------
  note: - Vdc--------------------------
  note: N -----------
  note: |
      | |
      | |
      | |
      | |
      | |
      | |
      | |
      | |
      | |
      | |
  note: ---------- A
  note: ----------[D]---------
  note: ----------[D]---------
  note: |
      | |
      | [Q4]
      | |
      | |
      | |
  note: |
      | |
      | [Q3]
      | |
      | |
  note: |
      | |
      | [Q2]
      | |
      | |
  note: |
      | |
      | |
      | [Q1]
      | |
      | |
  note: 3-Phase, 3-Level
      | PWM Generator
  note: (B, C)
  note: 12: Q4 (phase C)
  note: 11: Q3 (phase C)
  note: 10: Q2 (phase C)
  note: 9: Q1 (phase C )
  note: 8: Q4 (phase B)
  note: 7: Q3 (phase B)
  note: 6: Q2 (phase B)
  note: 5: Q1 (phase B )
  note: 4: Q4 (phase A)
  note: 3: Q3 (phase A)
  note: 2: Q2 (phase A)
  note: 1: Q1 (phase A )
  note: Pulse Pattern
  Uref_abc : Inport
  Fsw : Inport  Port=2  PortDimensions=1
  Carriers Generator : Subsystem
  Relational Operator : RelationalOperator  OutDataTypeStr=float('double')  InputSameDT=on
  Relational Operator1 : RelationalOperator  Operator=<=  OutDataTypeStr=float('double')  InputSameDT=on
  State-to-Pulses Decoder : Subsystem
  Sum3 : Sum  Inputs=|+-  SaturateOnIntegerOverflow=on  InputSameDT=on  OutDataTypeStr=Inherit: Same as first input
  P : Outport
  wires:
  Uref_abc/1 -> Relational Operator1/1, Relational Operator/1
  State-to-Pulses Decoder/1(Pulses) -> P/1
  Relational Operator/1 -> Sum3/1
  Relational Operator1/1 -> Sum3/2
  Carriers Generator/1(C+) -> Relational Operator/2
  Carriers Generator/2(C-) -> Relational Operator1/2
  Fsw/1 -> Carriers Generator/1(Fsw)
  Sum3/1 -> State-to-Pulses Decoder/1(State)  "State (+1,0,-1)"

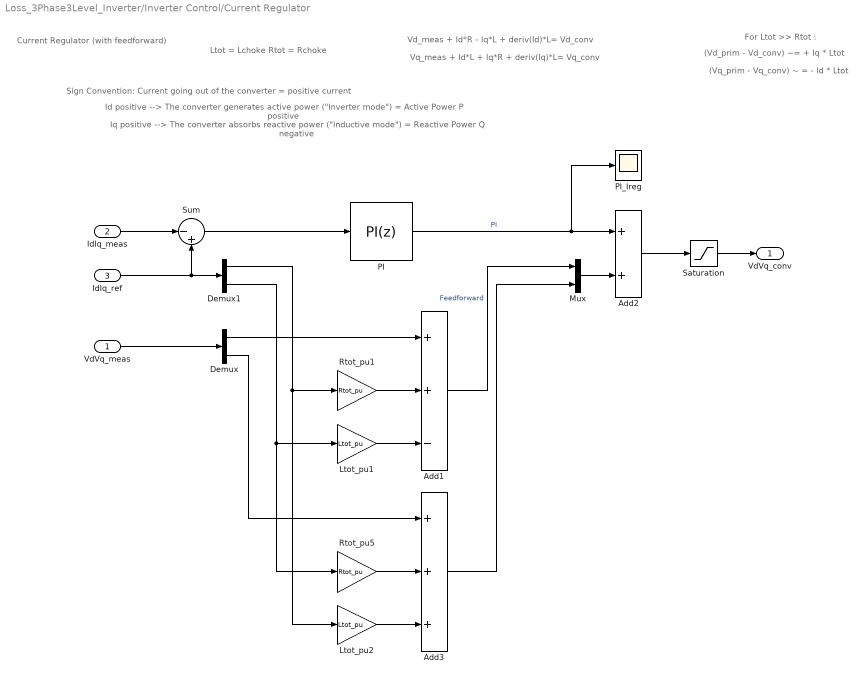
== system Loss_3Phase3Level_Inverter/Inverter Control/Current Regulator ==
  note: For Ltot >> Rtot :
  note: (Vq_prim - Vq_conv) ~ = - Id * Ltot
  note: (Vd_prim - Vd_conv) ~= + Iq * Ltot
  note: Ltot = Lchoke
      | Rtot = Rchoke
  note: Id positive --> The converter generates active power ("Inverter mode") = Active Power P positive
  note: Iq positive --> The converter absorbs reactive power ("Inductive mode") = Reactive Power Q negative
  note: Sign Convention: Current going out of the converter = positive current
  note: Current Regulator
      | (with feedforward)
  note: Vq_meas + Id*L + Iq*R + deriv(Iq)*L= Vq_conv
  note: Vd_meas + Id*R - Iq*L + deriv(Id)*L= Vd_conv
  VdVq_meas : Inport  PortDimensions=2
  IdIq_meas : Inport  Port=2  PortDimensions=2
  IdIq_ref : Inport  Port=3  PortDimensions=2
  Add1 : Sum  Inputs=++-
  Add2 : Sum
  Add3 : Sum  Inputs=+++
  Demux : Demux  Outputs=2
  Demux1 : Demux  Outputs=2
  Ltot_pu1 : Gain  Gain=Ltot_pu  SaturateOnIntegerOverflow=on  OutDataTypeStr=Inherit: Same as input  ParamDataTypeStr=Inherit: Same as input
  Ltot_pu2 : Gain  Gain=Ltot_pu  SaturateOnIntegerOverflow=on  OutDataTypeStr=Inherit: Same as input  ParamDataTypeStr=Inherit: Same as input
  Mux : Mux  Inputs=2
  PI : simulink/Continuous/PID Controller  Controller=PI  TimeDomain=Discrete-time  SampleTime=Ts  IntegratorMethod=Forward Euler  FilterMethod=Forward Euler  Form=Parallel  P=Kp_Ireg  I=Ki_Ireg  D=0  N=100  InitialConditionSource=internal  InitialConditionForIntegrator=0  InitialConditionForFilter=0  ExternalReset=none  LimitOutput=on  UpperSaturationLimit=2  LowerSaturationLimit=-2  LinearizeAsGain=off  AntiWindupMode=none  Kb=1  TrackingMode=off  Kt=1  PParamMin=[]  PParamMax=[]  IParamMin=[]  IParamMax=[]  DParamMin=[]  DParamMax=[]  NParamMin=[]  NParamMax=[]  KbParamMin=[]  KbParamMax=[]  KtParamMin=[]  KtParamMax=[]  POutMin=[]  POutMax=[]  IOutMin=[]  IOutMax=[]  DOutMin=[]  DOutMax=[]  NOutMin=[]  NOutMax=[]  KbOutMin=[]  KbOutMax=[]  KtOutMin=[]  KtOutMax=[]  IntegratorOutMin=[]  IntegratorOutMax=[]  FilterOutMin=[]  FilterOutMax=[]  SumOutMin=[]  SumOutMax=[]  SumI1OutMin=[]  SumI1OutMax=[]  SumI2OutMin=[]  SumI2OutMax=[]  SumI3OutMin=[]  SumI3OutMax=[]  SumDOutMin=[]  SumDOutMax=[]  SaturationOutMin=[]  SaturationOutMax=[]  IntegratorContinuousStateAttributes=''  IntegratorStateMustResolveToSignalObject=off  IntegratorRTWStateStorageClass=Auto  FilterContinuousStateAttributes=''  FilterStateMustResolveToSignalObject=off  FilterRTWStateStorageClass=Auto
  PI_Ireg : Scope
      settings: TimeRange=1  YMin=-0.7  YMax=0.15  Decimation=2
  Rtot_pu1 : Gain  Gain=Rtot_pu  SaturateOnIntegerOverflow=on  OutDataTypeStr=Inherit: Same as input  ParamDataTypeStr=Inherit: Same as input
  Rtot_pu5 : Gain  Gain=Rtot_pu  SaturateOnIntegerOverflow=on  OutDataTypeStr=Inherit: Same as input  ParamDataTypeStr=Inherit: Same as input
  Saturation : Saturate  UpperLimit=2  LowerLimit=-2
  Sum : Sum  Inputs=|-+
  VdVq_conv : Outport
  wires:
  Add3/1 -> Mux/2
  Demux/2 -> Add3/1
  Add1/1 -> Mux/1  "Feedforward"
  Ltot_pu2/1 -> Add3/3
  Rtot_pu5/1 -> Add3/2
  Demux1/2 -> Rtot_pu5/1, Ltot_pu1/1
  Ltot_pu1/1 -> Add1/3
  Demux1/1 -> Ltot_pu2/1, Rtot_pu1/1
  Rtot_pu1/1 -> Add1/2
  Demux/1 -> Add1/1
  VdVq_meas/1 -> Demux/1
  Saturation/1 -> VdVq_conv/1
  Add2/1 -> Saturation/1
  IdIq_meas/1 -> Sum/1
  IdIq_ref/1 -> Demux1/1, Sum/2
  Sum/1 -> PI/1
  PI/1 -> Add2/1, PI_Ireg/1  "PI"
  Mux/1 -> Add2/2

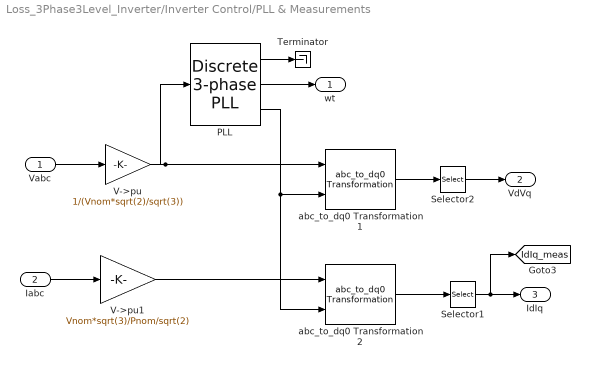
== system Loss_3Phase3Level_Inverter/Inverter Control/PLL & Measurements ==
  Vabc : Inport
  Iabc : Inport  Port=2
  PLL : powerlib_extras/Discrete  Control Blocks/Discrete 3-phase PLL  Fmin=45  Par_Init="[-0.57  Fnom]"  ParK=[60 1400]  Ts=Ts  AGC=off
  Selector1 : Selector  InputPortWidth=3  IndexOptions=Index vector (dialog)  Indices=[1 2]  OutputSizes=1
  Selector2 : Selector  InputPortWidth=3  IndexOptions=Index vector (dialog)  Indices=[1 2]  OutputSizes=1
  Terminator : Terminator
  V->pu : Gain  Gain=1/(Vnom*sqrt(2)/sqrt(3))  SaturateOnIntegerOverflow=on  OutDataTypeStr=Inherit: Same as input  ParamDataTypeStr=Inherit: Same as input
  V->pu1 : Gain  Gain=Vnom*sqrt(3)/Pnom/sqrt(2)  SaturateOnIntegerOverflow=on  OutDataTypeStr=Inherit: Same as input  ParamDataTypeStr=Inherit: Same as input
  abc_to_dq0 Transformation1 : powerlib_extras/Measurements/abc_to_dq0 Transformation
  abc_to_dq0 Transformation2 : powerlib_extras/Measurements/abc_to_dq0 Transformation
  wt : Outport
  VdVq : Outport  Port=2
  IdIq : Outport  Port=3
  tag scope: IdIq_meas=global
  wires:
  PLL/1 -> Terminator/1
  PLL/3 -> abc_to_dq0 Transformation1/2, abc_to_dq0 Transformation2/2
  Selector1/1 -> IdIq/1, [IdIq_meas]
  Selector2/1 -> VdVq/1
  abc_to_dq0 Transformation1/1 -> Selector2/1
  Iabc/1 -> V->pu1/1
  Vabc/1 -> V->pu/1
  PLL/2 -> wt/1
  abc_to_dq0 Transformation2/1 -> Selector1/1
  V->pu/1 -> abc_to_dq0 Transformation1/1, PLL/1
  V->pu1/1 -> abc_to_dq0 Transformation2/1

== system Loss_3Phase3Level_Inverter/Inverter Control/PQ Regulator ==
  PQ_meas : Inport
  PQ_ref : Inport  Port=2
  -1<Iq<+1 : Saturate  UpperLimit=1  LowerLimit=-1
  Add1 : Sum  Inputs=+-
  Discrete PI Controller : powerlib_extras/Discrete  Control Blocks/Discrete PI Controller  Kp=Kp_PQreg  Ki=Ki_PQreg  Par_Limits=[1 -1]  Init=0  Ts=Ts
  PQ->pu : Gain  Gain=1e3/Pnom  SaturateOnIntegerOverflow=on  OutDataTypeStr=Inherit: Same as input  ParamDataTypeStr=Inherit: Same as input
  PQ->pu1 : Gain  Gain="[ -1  +1 ]"  SaturateOnIntegerOverflow=on  OutDataTypeStr=Inherit: Same as input  ParamDataTypeStr=Inherit: Same as input
  IdIq_ref : Outport
  tag scope: IdIq_ref=global, PQmeas=global, PQref=global
  wires:
  Add1/1 -> PQ->pu/1
  Discrete PI Controller/1 -> -1<Iq<+1/1
  PQ->pu1/1 -> Discrete PI Controller/1
  PQ_meas/1 -> Add1/1, [PQmeas]
  -1<Iq<+1/1 -> IdIq_ref/1, [IdIq_ref]
  PQ_ref/1 -> Add1/2, [PQref]
  PQ->pu/1 -> PQ->pu1/1

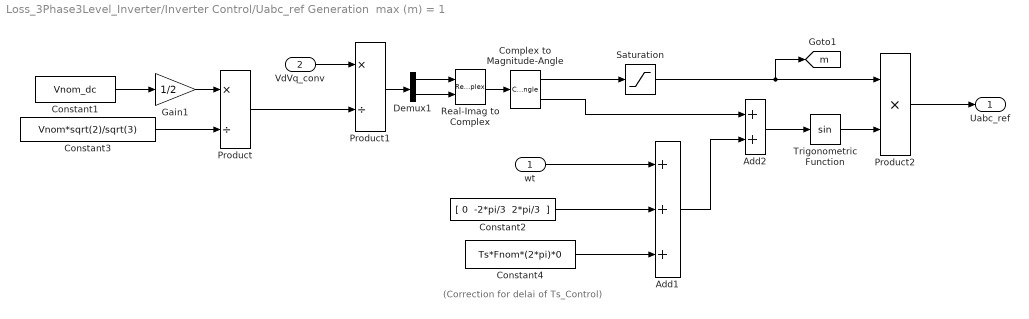
== system Loss_3Phase3Level_Inverter/Inverter Control/Uabc_ref Generation  max (m) = 1 ==
  note: (Correction for delai of Ts_Control)
  wt : Inport
  VdVq_conv : Inport  Port=2
  Add1 : Sum  Inputs=+++
  Add2 : Sum
  Complex to Magnitude-Angle : ComplexToMagnitudeAngle
  Constant1 : Constant  Value=Vnom_dc
  Constant2 : Constant  Value="[ 0  -2*pi/3  2*pi/3  ]"
  Constant3 : Constant  Value=Vnom*sqrt(2)/sqrt(3)
  Constant4 : Constant  Value=Ts*Fnom*(2*pi)*0
  Demux1 : Demux  Outputs=2
  Gain1 : Gain  Gain=1/2
  Product : Product  Inputs=*/  RndMeth=Zero
  Product1 : Product  Inputs=*/  RndMeth=Zero
  Product2 : Product  Inputs=**  RndMeth=Zero
  Real-Imag to Complex : RealImagToComplex
  Saturation : Saturate  UpperLimit=1  LowerLimit=0
  Trigonometric Function : Trigonometry
  Uabc_ref : Outport
  tag scope: m=global
  wires:
  Constant4/1 -> Add1/3
  wt/1 -> Add1/1
  Product2/1 -> Uabc_ref/1
  Trigonometric Function/1 -> Product2/2
  Add2/1 -> Trigonometric Function/1
  Add1/1 -> Add2/2
  Product/1 -> Product1/2
  Constant3/1 -> Product/2
  Constant2/1 -> Add1/2
  Demux1/2 -> Real-Imag to Complex/2
  Demux1/1 -> Real-Imag to Complex/1
  Real-Imag to Complex/1 -> Complex to Magnitude-Angle/1
  Gain1/1 -> Product/1
  Product1/1 -> Demux1/1
  VdVq_conv/1 -> Product1/1
  Constant1/1 -> Gain1/1
  Complex to Magnitude-Angle/1 -> Saturation/1
  Complex to Magnitude-Angle/2 -> Add2/1
  Saturation/1 -> Product2/1, [m]

== system Loss_3Phase3Level_Inverter/Simscape Heat Sink  Thermal Model/PS2S ==
  Add1 : Sum  Inputs=+-
  K1 : Constant  Value=273
  PS-Simulink Converter : nesl_utility/PS-Simulink Converter  PhysicalDomain=network_engine_domain  LeftPortType=input  RightPortType=output  SubClassName=ps_output  Unit=1  AffineConversion=off
  In : PMIOPort  Port=1  Side=Left
  Out : Outport
  wires:
  K1/1 -> Add1/2
  PS-Simulink Converter/1 -> Add1/1
  Add1/1 -> Out/1
  connections:
  In/RConn1 -- PS-Simulink Converter/LConn1

== system Loss_3Phase3Level_Inverter/Simscape Heat Sink  Thermal Model/S2PS1 ==
  In : Inport
  Add : Sum
  K2 : Constant  Value=273
  Simulink-PS Converter : nesl_utility/Simulink-PS Converter  PhysicalDomain=network_engine_domain  LeftPortType=input  RightPortType=output  SubClassName=ps_input  Unit=1  AffineConversion=off  InputFilterTimeConstant=1e-4  UdotUserProvided=0  SimscapeFilterOrder=1  InputFiltering=off
  Out : PMIOPort  Port=1  Side=Right
  wires:
  Add/1 -> Simulink-PS Converter/1
  K2/1 -> Add/1
  In/1 -> Add/2
  connections:
  Out/RConn1 -- Simulink-PS Converter/RConn1

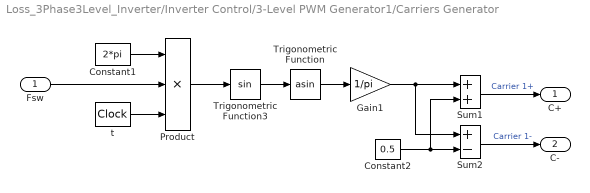
== system Loss_3Phase3Level_Inverter/Inverter Control/3-Level PWM Generator1/Carriers Generator ==
  Fsw : Inport
  Constant1 : Constant  Value=2*pi
  Constant2 : Constant  Value=0.5
  Gain1 : Gain  Gain=1/pi  SaturateOnIntegerOverflow=on  OutDataTypeStr=Inherit: Same as input  ParamDataTypeStr=Inherit: Same as input
  Product : Product  Inputs=3  SaturateOnIntegerOverflow=on  InputSameDT=on  OutDataTypeStr=Inherit: Same as first input
  Sum1 : Sum  SaturateOnIntegerOverflow=on  InputSameDT=on  OutDataTypeStr=Inherit: Same as first input
  Sum2 : Sum  Inputs=+-  SaturateOnIntegerOverflow=on  InputSameDT=on  OutDataTypeStr=Inherit: Same as first input
  Trigonometric Function : Trigonometry  Operator=asin
  Trigonometric Function3 : Trigonometry
  t : DigitalClock  SampleTime=Ts
  C+ : Outport
  C- : Outport  Port=2
  wires:
  Trigonometric Function/1 -> Gain1/1
  Trigonometric Function3/1 -> Trigonometric Function/1
  Gain1/1 -> Sum1/1, Sum2/1
  Constant2/1 -> Sum2/2, Sum1/2
  Sum2/1 -> C-/1  "Carrier 1-"
  Sum1/1 -> C+/1  "Carrier 1+"
  Constant1/1 -> Product/1
  Fsw/1 -> Product/2
  t/1 -> Product/3
  Product/1 -> Trigonometric Function3/1

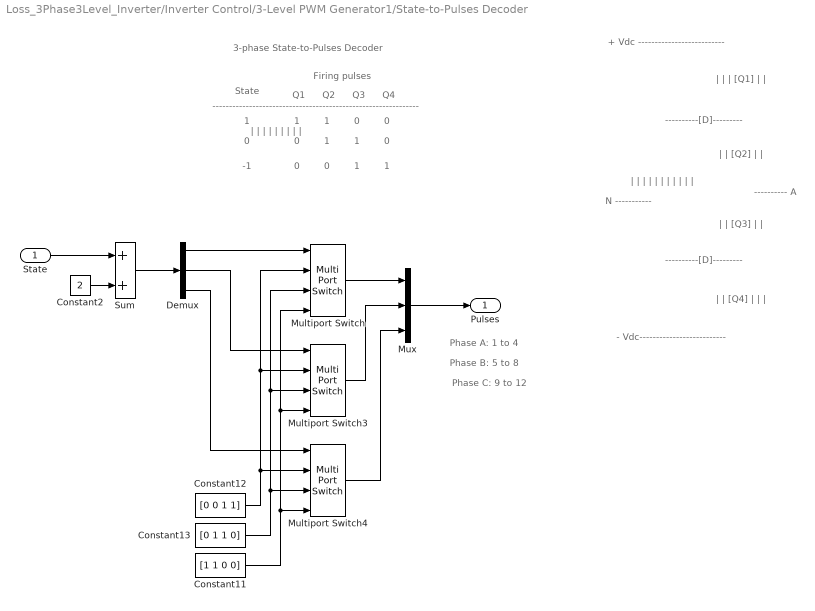
== system Loss_3Phase3Level_Inverter/Inverter Control/3-Level PWM Generator1/State-to-Pulses Decoder ==
  note: + Vdc --------------------------
  note: - Vdc--------------------------
  note: N -----------
  note: |
      | |
      | |
      | |
      | |
      | |
      | |
      | |
      | |
      | |
      | |
  note: ---------- A
  note: ----------[D]---------
  note: ----------[D]---------
  note: |
      | |
      | [Q4]
      | |
      | |
      | |
  note: |
      | |
      | [Q3]
      | |
      | |
  note: |
      | |
      | [Q2]
      | |
      | |
  note: |
      | |
      | |
      | [Q1]
      | |
      | |
  note: Phase C: 9 to 12
  note: Phase A: 1 to 4
  note: Phase B: 5 to 8
  note: 3-phase State-to-Pulses Decoder
  note: --------------------------------------------------------------
  note: |
      | |
      | |
      | |
      | |
      | |
      | |
      | |
      | |
  note: 1
  note: 1
  note: 0
  note: 0
  note: -1
  note: 0
  note: 1
  note: 1
  note: 0
  note: 0
  note: Q4
  note: Q3
  note: Q2
  note: Q1
  note: 0
  note: 0
  note: 1
  note: 1
  note: Firing pulses
  note: 1
  note: State
  State : Inport  PortDimensions=3
  Constant11 : Constant  Value=[1 1 0 0]
  Constant12 : Constant  Value=[0 0 1 1]
  Constant13 : Constant  Value=[0 1 1 0]
  Constant2 : Constant  Value=2
  Demux : Demux  Outputs=3
  Multiport Switch : MultiPortSwitch  zeroidx=off  InputSameDT=on
  Multiport Switch3 : MultiPortSwitch  zeroidx=off  InputSameDT=on
  Multiport Switch4 : MultiPortSwitch  zeroidx=off  InputSameDT=on
  Mux : Mux  Inputs=[4 4 4]
  Sum : Sum  SaturateOnIntegerOverflow=on  InputSameDT=on  OutDataTypeStr=Inherit: Same as first input
  Pulses : Outport
  wires:
  Multiport Switch4/1 -> Mux/3
  Multiport Switch3/1 -> Mux/2
  Multiport Switch/1 -> Mux/1
  Constant11/1 -> Multiport Switch4/4, Multiport Switch3/4, Multiport Switch/4
  Constant13/1 -> Multiport Switch4/3, Multiport Switch3/3, Multiport Switch/3
  Constant12/1 -> Multiport Switch4/2, Multiport Switch3/2, Multiport Switch/2
  Demux/3 -> Multiport Switch4/1
  Demux/2 -> Multiport Switch3/1
  Demux/1 -> Multiport Switch/1
  Constant2/1 -> Sum/2
  State/1 -> Sum/1
  Sum/1 -> Demux/1
  Mux/1 -> Pulses/1
